simulink model "ABS_simulink_model"  (R2022b)
settings: Solver=ode45  StartTime=0.0  StopTime=25  MaxStep=0.01  RelTol=1e-3  AbsTol=1e-6
values from neighbouring files (symbols this model uses):
  ctrl = 0    [ABS_model_script.m]
  g = 9.8    [ABS_model_script.m]
  I = 0.5*m*(R^2)    (= 0.453299)    [ABS_model_script.m]
  Kf = 1    [ABS_model_script.m]
  m = 22    [ABS_model_script.m]
  mu = [0 .4 .8 .97 1.0 .98 .96 .94 .92 .9 .88 .855 .83 .81 .79 .77 .75 .73 .72 .71 .7]    [ABS_model_script.m]
  R = 0.203    [ABS_model_script.m]
  slip = (0:.05:1.0)    [ABS_model_script.m]
  v0 = 25    [ABS_model_script.m]
settings Model: Creator=Arjun Rajan  LastModifiedBy=Arjun Rajan
settings SolverCC: AutoScaleAbsTol=off
settings DataIOCC: SaveFormat=Array  ReturnWorkspaceOutputs=off
settings ModelReferenceCC: EnableRefExpFcnMdlSchedulingChecks=on  PropagateSignalLabelsOutOfModel=off

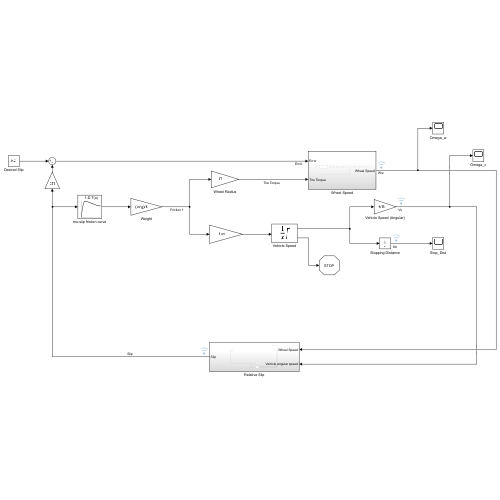
[thumbnail: Simulink's stored preview of the top-level diagram]
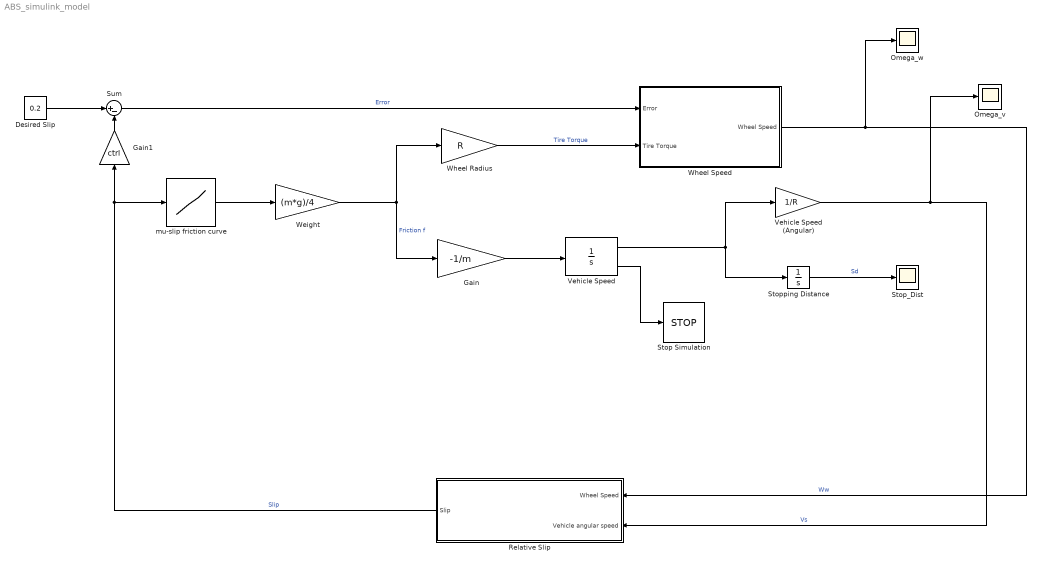
== system ABS_simulink_model ==
  Desired Slip : Constant  Value=0.2
  Gain : Gain  Gain=-1/m  SaturateOnIntegerOverflow=on  OutDataTypeStr=Inherit: Same as input  ParamDataTypeStr=Inherit: Same as input
  Gain1 : Gain  Gain=ctrl
  Omega_v : Scope
  Omega_w : Scope
  Relative Slip : Subsystem
  Stop Simulation : Stop
  Stop_Dist : Scope
  Stopping Distance : Integrator
  Sum : Sum  Inputs=|+-
  "Vehicle Speed " : Integrator  InitialCondition=v0  LimitOutput=on  UpperSaturationLimit=1000  LowerSaturationLimit=0  ShowSaturationPort=on
  Vehicle Speed (Angular) : Gain  Gain=1/R
  Weight : Gain  Gain=(m*g)/4  SaturateOnIntegerOverflow=on  OutDataTypeStr=Inherit: Same as input  ParamDataTypeStr=Inherit: Same as input
  Wheel Radius : Gain  Gain=R
  Wheel Speed : Subsystem
  mu-slip friction curve : Lookup_n-D  NumberOfTableDimensions=1  BreakpointsForDimension1=slip  Table=mu  SaturateOnIntegerOverflow=on
  wires:
  Desired Slip/1 -> Sum/1
  mu-slip friction curve/1 -> Weight/1
  Weight/1 -> Gain/1, Wheel Radius/1  "Friction f"
  Sum/1 -> Wheel Speed/1(Error)  "Error"
  Gain/1 -> "Vehicle Speed "/1
  "Vehicle Speed "/1 -> Vehicle Speed (Angular)/1, Stopping Distance/1
  "Vehicle Speed "/2 -> Stop Simulation/1
  Wheel Radius/1 -> Wheel Speed/2(Tire Torque)  "Tire Torque"
  Gain1/1 -> Sum/2
  Stopping Distance/1 -> Stop_Dist/1  "Sd"
  Relative Slip/1(Slip) -> mu-slip friction curve/1, Gain1/1  "Slip"
  Wheel Speed/1(Wheel Speed) -> Omega_w/1, Relative Slip/1(Wheel Speed)  "Ww"
  Vehicle Speed (Angular)/1 -> Omega_v/1, Relative Slip/2(Vehicle angular speed)  "Vs"

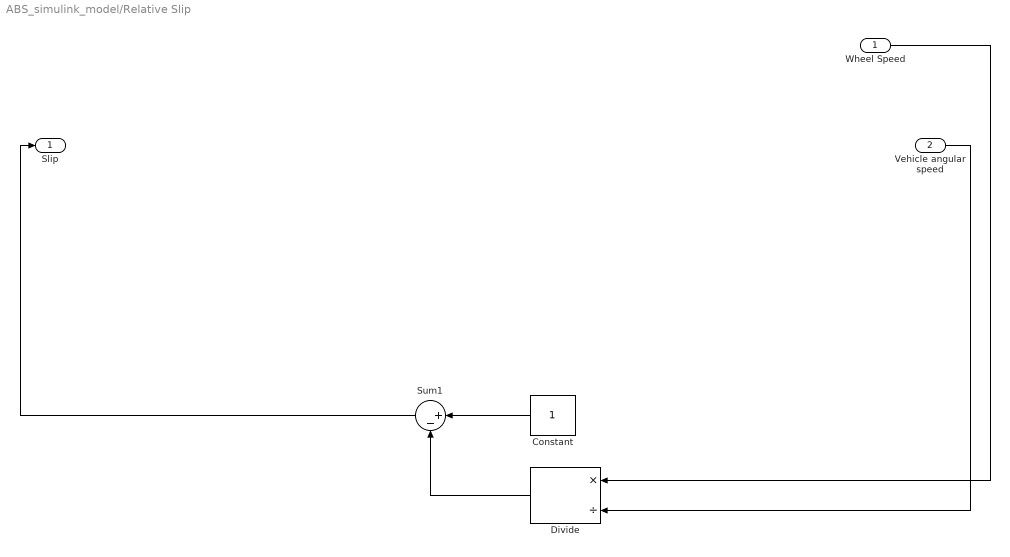
== system ABS_simulink_model/Relative Slip ==
  Wheel Speed : Inport
  Vehicle angular speed : Inport  Port=2
  Constant : Constant
  Divide : Product  Inputs=*/
  Sum1 : Sum  Inputs=|+-
  Slip : Outport
  wires:
  Constant/1 -> Sum1/1
  Divide/1 -> Sum1/2
  Sum1/1 -> Slip/1
  Wheel Speed/1 -> Divide/1
  Vehicle angular speed/1 -> Divide/2

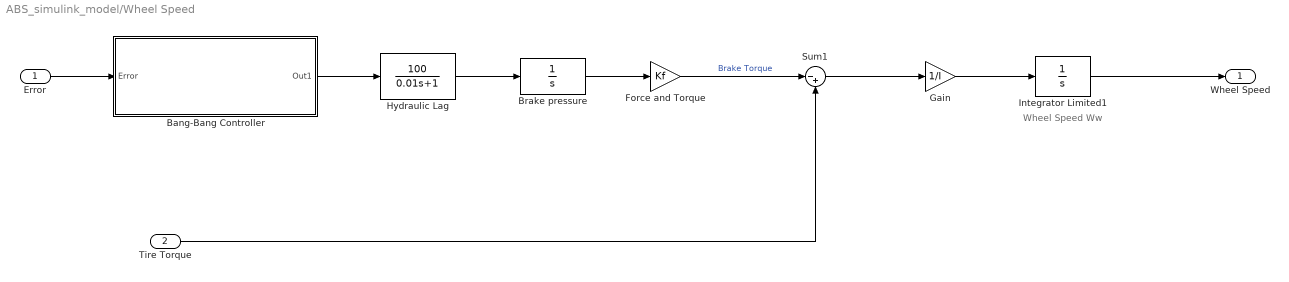
== system ABS_simulink_model/Wheel Speed ==
  note: Wheel Speed Ww
  Error : Inport
  Tire Torque : Inport  Port=2
  Bang-Bang Controller : Subsystem
  Brake pressure : Integrator  LimitOutput=on  UpperSaturationLimit=1500  LowerSaturationLimit=0
  Force and Torque : Gain  Gain=Kf  SaturateOnIntegerOverflow=on  OutDataTypeStr=Inherit: Same as input  ParamDataTypeStr=Inherit: Same as input
  Gain : Gain  Gain=1/I
  Hydraulic Lag : TransferFcn  Numerator=[100]  Denominator=[0.01 1]
  Integrator Limited1 : Integrator  InitialCondition=v0/R  LimitOutput=on  UpperSaturationLimit=1000  LowerSaturationLimit=0
  Sum1 : Sum  Inputs=|-+
  Wheel Speed : Outport
  wires:
  Hydraulic Lag/1 -> Brake pressure/1
  Gain/1 -> Integrator Limited1/1
  Tire Torque/1 -> Sum1/2
  Sum1/1 -> Gain/1
  Integrator Limited1/1 -> Wheel Speed/1
  Brake pressure/1 -> Force and Torque/1
  Force and Torque/1 -> Sum1/1  "Brake Torque"
  Bang-Bang Controller/1(Out1) -> Hydraulic Lag/1
  Error/1 -> Bang-Bang Controller/1(Error)

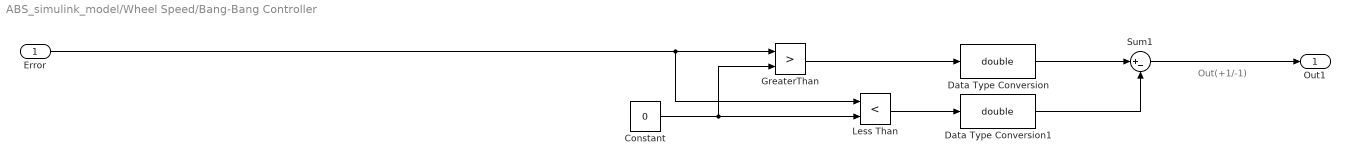
== system ABS_simulink_model/Wheel Speed/Bang-Bang Controller ==
  note: Out(+1/-1)
  Error : Inport
  Constant : Constant  Value=0
  Data Type Conversion : DataTypeConversion  OutDataTypeStr=double  SaturateOnIntegerOverflow=off
  Data Type Conversion1 : DataTypeConversion  OutDataTypeStr=double  SaturateOnIntegerOverflow=off
  GreaterThan : RelationalOperator  Operator=>  OutDataTypeStr=boolean  RndMeth=Simplest  InputSameDT=off
  Less Than : RelationalOperator  Operator=<  OutDataTypeStr=boolean  RndMeth=Simplest  InputSameDT=off
  Sum1 : Sum  Inputs=|+-
  Out1 : Outport
  wires:
  Less Than/1 -> Data Type Conversion1/1
  Error/1 -> Less Than/1, GreaterThan/1
  GreaterThan/1 -> Data Type Conversion/1
  Constant/1 -> Less Than/2, GreaterThan/2
  Sum1/1 -> Out1/1
  Data Type Conversion1/1 -> Sum1/2
  Data Type Conversion/1 -> Sum1/1
